simulink model "EHB_MOTOR_r2018b"  (R2018b)
settings: Solver=FixedStepDiscrete  StartTime=0.0  StopTime=0.2  FixedStep=0.0001  RelTol=1e-3  EnableMultiTasking=on
undefined symbols (not defined in the file): CAN_EHB_VCU0x125, CAN_EHB_VCU0x126, CAN_id0x120_Data, Cos_Table, Cos_Table1, EHB_DTC_status, Sin_BreakPoint, Sin_BreakPoint1, Sin_Table, Sin_Table1
libraries: simulink x30
(part 1 of 7)
settings Model: Creator=dell  LastModifiedBy=Administrator
settings SolverCC: PositivePriorityOrder=on  AutoInsertRateTranBlk=on
settings DataIOCC: LimitDataPoints=on  SaveFormat=Structure
settings OptimizationCC: DefaultParameterBehavior=Inlined  UseDivisionForNetSlopeComputation=on  InlineInvariantSignals=on  ExpressionDepthLimit=2147483647  ZeroExternalMemoryAtStartup=off  NoFixptDivByZeroProtection=on  EfficientFloat2IntCast=on  LifeSpan=1  MaxStackSize=64
settings DebuggingCC: CheckSSInitialOutputMsg=off  UnderspecifiedInitializationDetection=Classic  MergeDetectMultiDrivingBlocksExec=none  SignalResolutionControl=TryResolveAll  SolverPrmCheckMsg=warning  ParameterOverflowMsg=none  ParameterPrecisionLossMsg=none  FcnCallInpInsideContextMsg=warning  AssertControl=EnableAll  StateNameClashWarn=warning  SFUnexpectedBacktrackingDiag=warning  SFNoUnconditionalDefaultTransitionDiag=warning  SFExecutionAtInitializationDiag=none
settings HardwareCC: ProdBitPerPointer=32  ProdBitPerSizeT=32  ProdBitPerPtrDiffT=32  ProdLargestAtomicInteger=Integer  ProdLargestAtomicFloat=None  ProdIntDivRoundTo=Undefined  ProdEndianess=Unspecified  ProdWordSize=32  ProdHWDeviceType=Generic->32-bit Embedded Processor  TargetBitPerPointer=64  TargetBitPerSizeT=64  TargetBitPerPtrDiffT=64  TargetLargestAtomicInteger=Integer  TargetLongLongMode=on  TargetIntDivRoundTo=Zero  TargetEndianess=LittleEndian  TargetWordSize=64  TargetHWDeviceType=MATLAB Host  ProdEqTarget=off
settings ModelReferenceCC: UpdateModelReferenceTargets=IfOutOfDate  PropagateSignalLabelsOutOfModel=off
settings SFSimCC: SimUseLocalCustomCode=off  MATLABDynamicMemAlloc=off
settings SFSimCC: SimCustomHeaderCode=|
  | #define MCU_IDLE_ST     0
  | #define MCU_INIT_ST     1
  | #define MCU_START_ST    2
  | #define MCU_RUN_ST      3
  | #define MCU_FAULT_ST    4
  | #define MCU_WAIT_ST     5
  | 
  | // MCU_IDLE_ST = 0;
  | // MCU_INIT_ST = 1;
  | // MCU_START_ST = 2;
  | // MCU_RUN_ST = 3;
  | // MCU_FAULT_ST = 4;
  | // MCU_WAIT_ST = 5;
settings RTWCC: SystemTargetFile=ert.tlc  TemplateMakefile=ert_default_tmf  RTWUseLocalCustomCode=off  RTWUseSimCustomCode=on  IncludeHyperlinkInReport=on
settings RTWCC: CustomHeaderCode=|
  | #define MCU_IDLE_ST     0
  | #define MCU_INIT_ST     1
  | #define MCU_START_ST    2
  | #define MCU_RUN_ST      3
  | #define MCU_FAULT_ST    4
  | #define MCU_WAIT_ST     5
  | 
  | // MCU_IDLE_ST = 0;
  | // MCU_INIT_ST = 1;
  | // MCU_START_ST = 2;
  | // MCU_RUN_ST = 3;
  | // MCU_FAULT_ST = 4;
  | // MCU_WAIT_ST = 5;
settings CodeAppCC: GenerateComments=off  IgnoreCustomStorageClasses=off  CustomSymbolStrType=$N$R$M  SimulinkBlockComments=off  MATLABSourceComments=on  InternalIdentifier=Classic
settings ERTTargetCC: MultiwordLength=2048  IncludeFileDelimiter=UseQuote  InlinedParameterPlacement=NonHierarchical  ERTCustomFileTemplate=example_file_process.tlc  GlobalDataDefinition=InSeparateSourceFile  DataDefinitionFile=EHB_MOTOR_data.c  GlobalDataReference=InSeparateHeaderFile  ERTFilePackagingFormat=CompactWithDataFile  DataReferenceFile=EHB_MOTOR.h  ConvertIfToSwitch=off  SuppressUnreachableDefaultCases=off  IndentStyle=Allman  IndentSize=4  MemSecPackage=mpt
settings ConfigComp: CovMetricSettings=dw  CovSaveCumulativeToWorkspaceVar=on  CovSaveSingleToWorkspaceVar=on  CovExternalEMLEnable=off  CovSFcnEnable=off
settings SimscapeCC: SimscapeNormalizeSystem=off
settings ConfigurationSet: Description=SimMechanics 2G

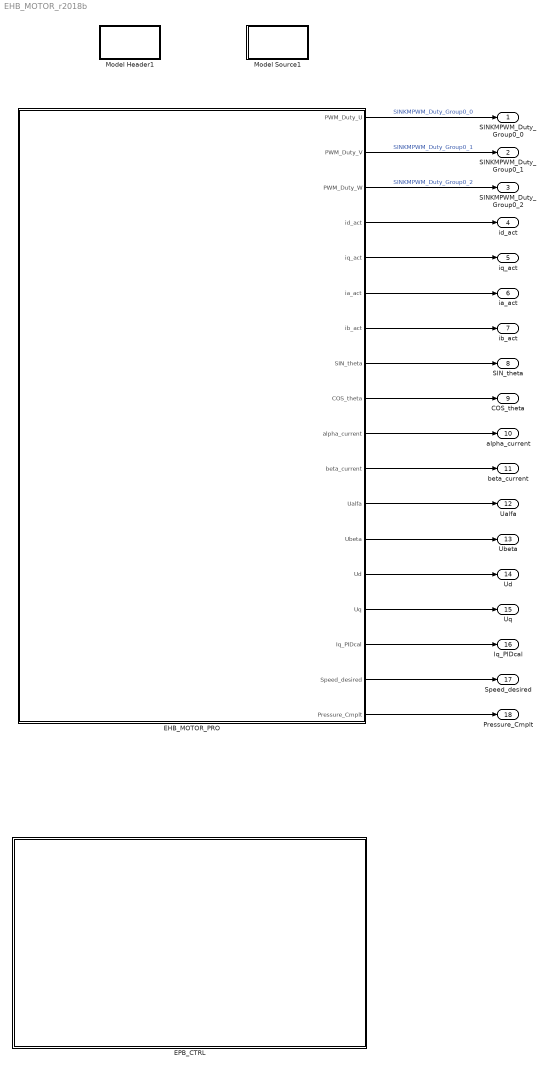
== system EHB_MOTOR_r2018b ==
  EHB_MOTOR_PRO : Subsystem  TreatAsAtomicUnit=on  RTWFcnName=isr_can_rx
      settings: MinAlgLoopOccurrences=on
  EPB_CTRL : Subsystem
  Model Header1 : Subsystem  mask(Model Header){ShowInLibBrowser=0}
      mask prompts: ShowInLibBrowser "Simulink:masks:CustCodeMaskParam1_MP"
      settings: CopyFcn=cccopyfcn(gcb)  OpenFcn=ccopenfcn('Model Header')
      mask Help: eval('feval(''rtwprivate'',''rtwhelpview'',''rtw_model_header_block'')');
      mask Display: disp('Model\nHeader');
  Model Source1 : Subsystem  mask(Model Source){ShowInLibBrowser=0}
      mask prompts: ShowInLibBrowser "Simulink:masks:CustCodeMaskParam1_MP"
      settings: CopyFcn=cccopyfcn(gcb)  OpenFcn=ccopenfcn('Model Source')
      mask Help: eval('feval(''rtwprivate'',''rtwhelpview'',''rtw_model_source_block'')');
      mask Display: disp('Model\nSource');
  SINKMPWM_Duty_Group0_0 : Outport
  SINKMPWM_Duty_Group0_1 : Outport  Port=2
  SINKMPWM_Duty_Group0_2 : Outport  Port=3
  id_act : Outport  Port=4
  iq_act : Outport  Port=5
  ia_act : Outport  Port=6
  ib_act : Outport  Port=7
  SIN_theta : Outport  Port=8
  COS_theta : Outport  Port=9
  alpha_current : Outport  Port=10  OutDataTypeStr=single
  beta_current : Outport  Port=11  OutDataTypeStr=single
  Ualfa : Outport  Port=12
  Ubeta : Outport  Port=13
  Ud : Outport  Port=14
  Uq : Outport  Port=15
  Iq_PIDcal : Outport  Port=16
  Speed_desired : Outport  Port=17
  Pressure_Cmplt : Outport  Port=18
  wires:
  EHB_MOTOR_PRO/18(Pressure_Cmplt) -> Pressure_Cmplt/1
  EHB_MOTOR_PRO/4(id_act) -> id_act/1
  EHB_MOTOR_PRO/7(ib_act) -> ib_act/1
  EHB_MOTOR_PRO/16(Iq_PIDcal) -> Iq_PIDcal/1
  EHB_MOTOR_PRO/11(beta_current) -> beta_current/1
  EHB_MOTOR_PRO/15(Uq) -> Uq/1
  EHB_MOTOR_PRO/5(iq_act) -> iq_act/1
  EHB_MOTOR_PRO/13(Ubeta) -> Ubeta/1
  EHB_MOTOR_PRO/3(PWM_Duty_W) -> SINKMPWM_Duty_Group0_2/1  "SINKMPWM_Duty_Group0_2"
  EHB_MOTOR_PRO/17(Speed_desired) -> Speed_desired/1
  EHB_MOTOR_PRO/8(SIN_theta) -> SIN_theta/1
  EHB_MOTOR_PRO/6(ia_act) -> ia_act/1
  EHB_MOTOR_PRO/9(COS_theta) -> COS_theta/1
  EHB_MOTOR_PRO/14(Ud) -> Ud/1
  EHB_MOTOR_PRO/10(alpha_current) -> alpha_current/1
  EHB_MOTOR_PRO/2(PWM_Duty_V) -> SINKMPWM_Duty_Group0_1/1  "SINKMPWM_Duty_Group0_1"
  EHB_MOTOR_PRO/12(Ualfa) -> Ualfa/1
  EHB_MOTOR_PRO/1(PWM_Duty_U) -> SINKMPWM_Duty_Group0_0/1  "SINKMPWM_Duty_Group0_0"

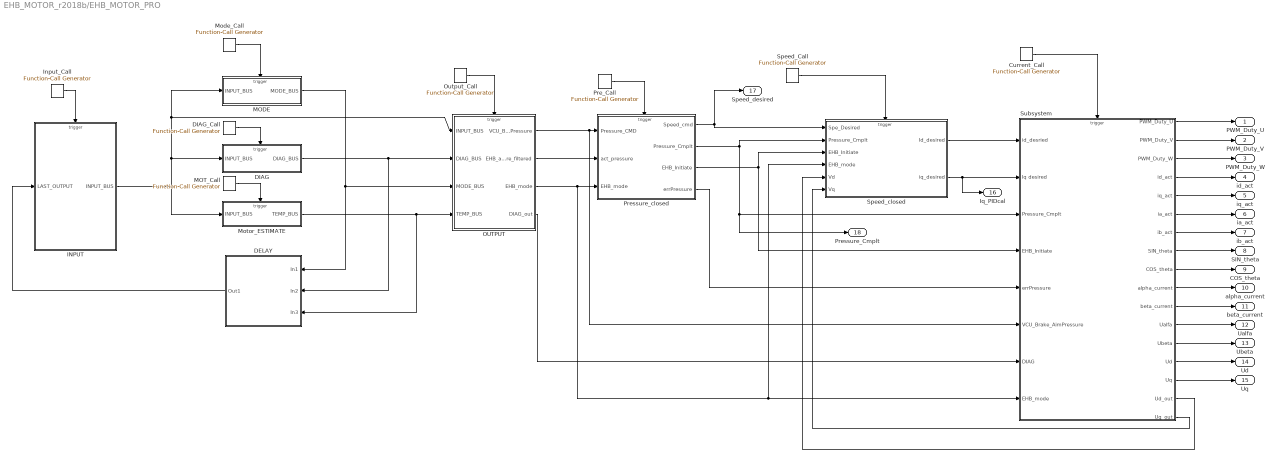
== system EHB_MOTOR_r2018b/EHB_MOTOR_PRO ==
  Current_Call : simulink/Ports & Subsystems/Function-Call Generator  sample_time=0.2  numberOfIterations=1
  DELAY : Subsystem
  DIAG : Subsystem
  DIAG_Call : simulink/Ports & Subsystems/Function-Call Generator  sample_time=0.01  numberOfIterations=1
  INPUT : Subsystem
  "Input_Call " : simulink/Ports & Subsystems/Function-Call Generator  sample_time=0.01  numberOfIterations=1
  MODE : Subsystem
  MOT_Call : simulink/Ports & Subsystems/Function-Call Generator  sample_time=0.01  numberOfIterations=1
  Mode_Call : simulink/Ports & Subsystems/Function-Call Generator  sample_time=0.01  numberOfIterations=1
  Motor_ESTIMATE : Subsystem
  OUTPUT : Subsystem
  Output_Call : simulink/Ports & Subsystems/Function-Call Generator  sample_time=0.01  numberOfIterations=1
  Pre_Call : simulink/Ports & Subsystems/Function-Call Generator  sample_time=0.05  numberOfIterations=1
  Pressure_closed : Subsystem
  "Speed_Call " : simulink/Ports & Subsystems/Function-Call Generator  sample_time=0.1  numberOfIterations=1
  Speed_closed : Subsystem
  Subsystem : Subsystem
  PWM_Duty_U : Outport
  PWM_Duty_V : Outport  Port=2
  PWM_Duty_W : Outport  Port=3
  id_act : Outport  Port=4
  iq_act : Outport  Port=5
  ia_act : Outport  Port=6  OutDataTypeStr=single
  ib_act : Outport  Port=7  OutDataTypeStr=single
  SIN_theta : Outport  Port=8
  COS_theta : Outport  Port=9
  alpha_current : Outport  Port=10  OutDataTypeStr=single
  beta_current : Outport  Port=11  OutDataTypeStr=single
  Ualfa : Outport  Port=12
  Ubeta : Outport  Port=13
  Ud : Outport  Port=14
  Uq : Outport  Port=15
  Iq_PIDcal : Outport  Port=16
  Speed_desired : Outport  Port=17
  Pressure_Cmplt : Outport  Port=18
  wires:
  "Speed_Call "/1 -> Speed_closed/Trigger
  Pressure_closed/1(Speed_cmd) -> Speed_closed/1(Spe_Desired), Speed_desired/1
  Subsystem/1(PWM_Duty_U) -> PWM_Duty_U/1
  Subsystem/2(PWM_Duty_V) -> PWM_Duty_V/1
  Subsystem/3(PWM_Duty_W) -> PWM_Duty_W/1
  Subsystem/4(id_act) -> id_act/1
  Subsystem/5(iq_act) -> iq_act/1
  Subsystem/6(ia_act) -> ia_act/1
  Subsystem/7(ib_act) -> ib_act/1
  Subsystem/8(SIN_theta) -> SIN_theta/1
  Subsystem/9(COS_theta) -> COS_theta/1
  Subsystem/10(alpha_current) -> alpha_current/1
  Subsystem/11(beta_current) -> beta_current/1
  Subsystem/12(Ualfa) -> Ualfa/1
  Subsystem/13(Ubeta) -> Ubeta/1
  Subsystem/14(Ud) -> Ud/1
  Subsystem/15(Uq) -> Uq/1
  Current_Call/1 -> Subsystem/Trigger
  Speed_closed/2(iq_desired) -> Iq_PIDcal/1, Subsystem/2(Iq desired)
  OUTPUT/1(VCU_Brake_AimPressure) -> Pressure_closed/1(Pressure_CMD), Subsystem/6(VCU_Brake_AimPressure)
  Pressure_closed/4(errPressure) -> Subsystem/5(errPressure)
  Pressure_closed/2(Pressure_Cmplt) -> Speed_closed/2(Pressure_Cmplt), Pressure_Cmplt/1, Subsystem/3(Pressure_Cmplt)
  OUTPUT/4(DIAG_out) -> Subsystem/7(DIAG)
  Pressure_closed/3(EHB_Initiate) -> Speed_closed/3(EHB_Initiate), Subsystem/4(EHB_Initiate)
  Pre_Call/1 -> Pressure_closed/Trigger
  "Input_Call "/1 -> INPUT/Trigger
  DIAG/1(DIAG_BUS) -> DELAY/2(In2), OUTPUT/2(DIAG_BUS)
  Motor_ESTIMATE/1(TEMP_BUS) -> DELAY/3(In3), OUTPUT/4(TEMP_BUS)
  MODE/1(MODE_BUS) -> DELAY/1(In1), OUTPUT/3(MODE_BUS)
  DELAY/1(Out1) -> INPUT/1(LAST_OUTPUT)
  OUTPUT/2(EHB_actPressure_filtered) -> Pressure_closed/2(act_pressure)
  INPUT/1(INPUT_BUS) -> MODE/1(INPUT_BUS), OUTPUT/1(INPUT_BUS), DIAG/1(INPUT_BUS), Motor_ESTIMATE/1(INPUT_BUS)
  Speed_closed/1(Id_desired) -> Subsystem/1(id_desried)
  Mode_Call/1 -> MODE/Trigger
  DIAG_Call/1 -> DIAG/Trigger
  Output_Call/1 -> OUTPUT/Trigger
  MOT_Call/1 -> Motor_ESTIMATE/Trigger
  OUTPUT/3(EHB_mode) -> Pressure_closed/3(EHB_mode), Speed_closed/4(EHB_mode), Subsystem/8(EHB_mode)
  Subsystem/17(Uq_out) -> Speed_closed/6(Vq)
  Subsystem/16(Ud_out) -> Speed_closed/5(Vd)

== system EHB_MOTOR_r2018b/EPB_CTRL ==
  Data Store Memory : DataStoreMemory  DataStoreName=EPB_PWMout  ReadBeforeWriteMsg=warning  WriteAfterWriteMsg=warning  WriteAfterReadMsg=warning  ShowAdditionalParam=off  OutDataTypeStr=uint16
      settings: RTWStateStorageClass=ExportedGlobal
  Data Store Memory1 : DataStoreMemory  DataStoreName=EPB_state  ReadBeforeWriteMsg=warning  WriteAfterWriteMsg=warning  WriteAfterReadMsg=warning  ShowAdditionalParam=off  OutDataTypeStr=uint8
      settings: RTWStateStorageClass=ExportedGlobal
  Data Store Memory2 : DataStoreMemory  DataStoreName=EPB_CMD  ReadBeforeWriteMsg=warning  WriteAfterWriteMsg=warning  WriteAfterReadMsg=warning  ShowAdditionalParam=off  OutDataTypeStr=uint8
      settings: RTWStateStorageClass=ExportedGlobal
  Data Store Memory3 : DataStoreMemory  DataStoreName=Clamp_ok  ReadBeforeWriteMsg=warning  WriteAfterWriteMsg=warning  WriteAfterReadMsg=warning  ShowAdditionalParam=off  OutDataTypeStr=boolean
      settings: RTWStateStorageClass=ExportedGlobal
  Data Store Memory4 : DataStoreMemory  DataStoreName=Release_ok  ReadBeforeWriteMsg=warning  WriteAfterWriteMsg=warning  WriteAfterReadMsg=warning  ShowAdditionalParam=off  OutDataTypeStr=boolean
      settings: RTWStateStorageClass=ExportedGlobal
  Data Store Read : DataStoreRead  DataStoreName=EPB_CMD  DataStoreElements=EPB_CMD
  Data Store Write : DataStoreWrite  DataStoreName=EPB_PWMout  DataStoreElements=EPB_PWMout
  Data Store Write1 : DataStoreWrite  DataStoreName=EPB_state  DataStoreElements=EPB_state
  Data Store Write2 : DataStoreWrite  DataStoreName=Clamp_ok  DataStoreElements=Clamp_ok
  Data Store Write3 : DataStoreWrite  DataStoreName=Release_ok  DataStoreElements=Release_ok
  EPBDiag_Call : simulink/Ports & Subsystems/Function-Call Generator  sample_time=0.3  numberOfIterations=1
  EPBInput_Call : simulink/Ports & Subsystems/Function-Call Generator  sample_time=0.3  numberOfIterations=1
  EPB_CTRL : Subsystem
  EPB_Diag : Subsystem
  EPBctrl_Call : simulink/Ports & Subsystems/Function-Call Generator  sample_time=0.3  numberOfIterations=1
  Subsystem1 : Subsystem
  wires:
  EPB_Diag/1(EPB_DiagBUS) -> EPB_CTRL/2(EPB_DiagBUS)
  Subsystem1/1(EPB_INPUTBUS) -> EPB_Diag/1(In1), EPB_CTRL/3(EPB_INPUTBUS)
  EPBInput_Call/1 -> Subsystem1/Trigger
  EPB_CTRL/2(EPB_state) -> Data Store Write1/1
  EPB_CTRL/4(Release_ok) -> Data Store Write3/1
  EPBctrl_Call/1 -> EPB_CTRL/Trigger
  EPB_CTRL/1(EPB_PWMout) -> Data Store Write/1
  Data Store Read/1 -> EPB_CTRL/1(EPB_CMD)
  EPB_CTRL/3(Clamp_ok) -> Data Store Write2/1
  EPBDiag_Call/1 -> EPB_Diag/Trigger

== system EHB_MOTOR_r2018b/Model Header1 ==

== system EHB_MOTOR_r2018b/Model Source1 ==

== system EHB_MOTOR_r2018b/EHB_MOTOR_PRO/DELAY ==
  In1 : Inport
  In2 : Inport  Port=2
  In3 : Inport  Port=3
  Bus Creator : BusCreator  Inputs=3
  Unit Delay : UnitDelay  SampleTime=-1
  Unit Delay1 : UnitDelay  SampleTime=-1
  Unit Delay2 : UnitDelay  SampleTime=-1
  Out1 : Outport
  wires:
  In1/1 -> Unit Delay/1
  In2/1 -> Unit Delay1/1
  Unit Delay/1 -> Bus Creator/1  "MODE_DELAY"
  Unit Delay1/1 -> Bus Creator/2  "DIAG_DELAY"
  Unit Delay2/1 -> Bus Creator/3  "TEMP_DELAY"
  Bus Creator/1 -> Out1/1
  In3/1 -> Unit Delay2/1

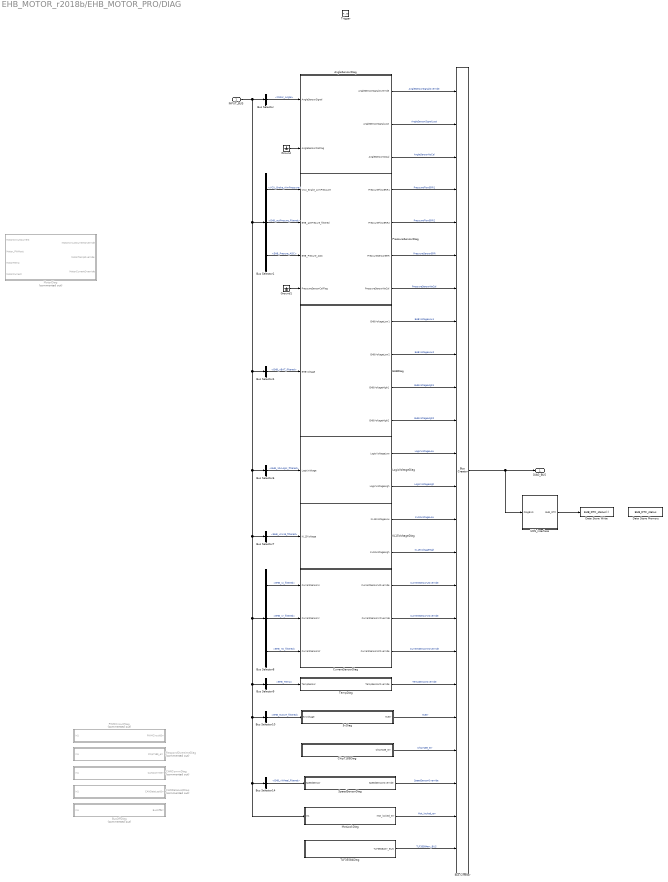
== system EHB_MOTOR_r2018b/EHB_MOTOR_PRO/DIAG ==
  INPUT_BUS : Inport
  Trigger : TriggerPort  TriggerType=function-call  VariantControl=Variant  PortDimensions=1
  5vDiag : Subsystem
  AngleSensorDiag : Subsystem
  Bus Creator : BusCreator  Inputs=24
  Bus Selector : BusSelector  OutputSignals=MOT_BUS.Motor_Angle
  Bus Selector1 : BusSelector  OutputSignals=CAN_BUS.VCU_Brake_AimPressure,AI_BUS.EHB_actPresure_filtered,AI_BUS.EHB_Presure_ADC
  Bus Selector10 : BusSelector  OutputSignals=AI_BUS.EHB_5vOUT_filtered
  Bus Selector14 : BusSelector  OutputSignals=AI_BUS.EHB_vWheel_filtered
  Bus Selector4 : BusSelector  OutputSignals=AI_BUS.EHB_vBAT_filtered
  Bus Selector6 : BusSelector  OutputSignals=AI_BUS.EHB_12vLogic_filtered
  Bus Selector7 : BusSelector  OutputSignals=AI_BUS.EHB_vKL15_filtered
  Bus Selector8 : BusSelector  OutputSignals=AI_BUS.EHB_iU_filtered,AI_BUS.EHB_iV_filtered,AI_BUS.EHB_iW_filtered
  Bus Selector9 : BusSelector  OutputSignals=AI_BUS.EHB_Temp
  BusOffDiag : Subsystem  Commented=on
  CANCommDiag : Subsystem  Commented=on
  CANDataLostDiag : Subsystem  Commented=on
  Chip7189Diag : Subsystem
  CurrentSensorDiag : Subsystem
  Data Store Memory : DataStoreMemory  DataStoreName=EHB_DTC_status  ReadBeforeWriteMsg=warning  WriteAfterWriteMsg=warning  WriteAfterReadMsg=warning  ShowAdditionalParam=off  OutDataTypeStr=uint8  Dimensions=50
      settings: RTWStateStorageClass=ExportedGlobal
  Data Store Write : DataStoreWrite  DataStoreName=EHB_DTC_status  DataStoreElements=EHB_DTC_status(:)
  EHBDiag : Subsystem
  Ground : Ground
  Ground1 : Ground
  KL15VoltageDiag : Subsystem
  LogicVoltageDiag : Subsystem
  MotLockDiag : Subsystem
  MotorDiag : Subsystem  Commented=on
  PWMCircuitDiag : Subsystem  Commented=on
  PressureSensorDiag : Subsystem
  RespondOvertimeDiag : Subsystem  Commented=on
  SpeedSensorDiag : Subsystem
  TLF35584Diag : Subsystem
  TempDiag : Subsystem
  UDS_interface : Subsystem
  DIAG_BUS : Outport
  wires:
  Bus Creator/1 -> DIAG_BUS/1, UDS_interface/1(DiagBUS)
  INPUT_BUS/1 -> Bus Selector14/1, MotLockDiag/1(In1), Bus Selector10/1, Bus Selector9/1, Bus Selector8/1, Bus Selector7/1, Bus Selector6/1, Bus Selector4/1, Bus Selector1/1, Bus Selector/1
  AngleSensorDiag/1(AngleSensorSignalOverride) -> Bus Creator/1  "AngleSensorSignalOverride"
  AngleSensorDiag/2(AngleSensorSignalLost) -> Bus Creator/2  "AngleSensorSignalLost"
  AngleSensorDiag/3(AngleSensorNoCal) -> Bus Creator/3  "AngleSensorNoCal"
  PressureSensorDiag/1(PressureFlowERR1) -> Bus Creator/4  "PressureFlowERR1"
  PressureSensorDiag/3(PressureSensorERR) -> Bus Creator/6  "PressureSensorERR"
  PressureSensorDiag/4(PressureSensorNoCal) -> Bus Creator/7  "PressureSensorNoCal"
  Bus Selector/1 -> AngleSensorDiag/1(AngleSensorSignal)  "<Motor_Angle>"
  Bus Selector1/2 -> PressureSensorDiag/2(EHB_actPresure_filtered)  "<EHB_actPresure_filtered>"
  EHBDiag/1(EHBVoltageLow1) -> Bus Creator/8  "EHBVoltageLow1"
  EHBDiag/3(EHBVoltageHigh1) -> Bus Creator/10  "EHBVoltageHigh1"
  Bus Selector4/1 -> EHBDiag/1(EHBVoltage)  "<EHB_vBAT_filtered>"
  LogicVoltageDiag/1(LogicVoltageLow) -> Bus Creator/12  "LogicVoltageLow"
  LogicVoltageDiag/2(LogicVoltageHigh) -> Bus Creator/13  "LogicVoltageHigh"
  Bus Selector6/1 -> LogicVoltageDiag/1(LogicVoltage)  "<EHB_12vLogic_filtered>"
  KL15VoltageDiag/1(KL15VoltageLow) -> Bus Creator/14  "KL15VoltageLow"
  KL15VoltageDiag/2(KL15VoltageHigh) -> Bus Creator/15  "KL15VoltageHigh"
  Bus Selector7/1 -> KL15VoltageDiag/1(KL15Voltage)  "<EHB_vKL15_filtered>"
  CurrentSensorDiag/1(CurrentSensorUOverride) -> Bus Creator/16  "CurrentSensorUOverride"
  CurrentSensorDiag/2(CurrentSensorVOverride) -> Bus Creator/17  "CurrentSensorVOverride"
  CurrentSensorDiag/3(CurrentSensorWOverride) -> Bus Creator/18  "CurrentSensorWOverride"
  Bus Selector8/1 -> CurrentSensorDiag/1(CurrentSensorU)  "<EHB_iU_filtered>"
  Bus Selector8/2 -> CurrentSensorDiag/2(CurrentSensorV)  "<EHB_iV_filtered>"
  TempDiag/1(TempSensorOverride) -> Bus Creator/19  "TempSensorOverride"
  Bus Selector9/1 -> TempDiag/1(TempSensor)  "<EHB_Temp>"
  Bus Selector10/1 -> 5vDiag/1(5vVoltage)  "<EHB_5vOUT_filtered>"
  5vDiag/1(5vErr) -> Bus Creator/20  "5vErr"
  Chip7189Diag/1(Chip7189_err) -> Bus Creator/21  "Chip7189_err"
  SpeedSensorDiag/1(SpeedSensorOverride) -> Bus Creator/22  "SpeedSensorOverride"
  Bus Selector14/1 -> SpeedSensorDiag/1(SpeedSensor)  "<EHB_vWheel_filtered>"
  Ground/1 -> AngleSensorDiag/2(AngleSensorCalFlag)
  Ground1/1 -> PressureSensorDiag/4(PressureSensorCalFlag)
  Bus Selector8/3 -> CurrentSensorDiag/3(CurrentSensorW)  "<EHB_iW_filtered>"
  Bus Selector1/1 -> PressureSensorDiag/1(VCU_Brake_AimPressure)  "<VCU_Brake_AimPressure>"
  PressureSensorDiag/2(PressureFlowERR2) -> Bus Creator/5  "PressureFlowERR2"
  EHBDiag/2(EHBVoltageLow2) -> Bus Creator/9  "EHBVoltageLow2"
  EHBDiag/4(EHBVoltageHigh2) -> Bus Creator/11  "EHBVoltageHigh2"
  MotLockDiag/1(Mot_locked_err) -> Bus Creator/23  "Mot_locked_err"
  Bus Selector1/3 -> PressureSensorDiag/3(EHB_Presure_ADC)  "<EHB_Presure_ADC>"
  UDS_interface/1(EHB_DTC) -> Data Store Write/1
  TLF35584Diag/1(TLF35584err_BUS) -> Bus Creator/24  "TLF35584err_BUS"

== system EHB_MOTOR_r2018b/EHB_MOTOR_PRO/INPUT ==
  LAST_OUTPUT : Inport
  Trigger : TriggerPort  TriggerType=function-call  VariantControl=Variant  PortDimensions=1
  AI : Subsystem
  Bus Creator : BusCreator  Inputs=5
  Bus Creator1 : BusCreator  Inputs=16
  Bus Creator2 : BusCreator  Inputs=5
  Bus Creator3 : BusCreator  Inputs=2
  Bus Creator4 : BusCreator  Inputs=10
  CAN : Subsystem
  DI : Subsystem
  MOTOR : Subsystem
  OUTPUT2INPUT : Subsystem
  INPUT_BUS : Outport
  wires:
  CAN/1(VCU_BrakingEnable) -> Bus Creator/1  "VCU_BrakingEnable"
  CAN/2(VCU_ParkingBrakeActive) -> Bus Creator/2  "VCU_ParkingBrakeActive"
  CAN/3(VCU_Brake_AimPressure) -> Bus Creator/3  "VCU_Brake_AimPressure"
  CAN/4(VCU_RollingCounter) -> Bus Creator/4  "VCU_RollingCounter"
  CAN/5(VCU_Checksum) -> Bus Creator/5  "VCU_Checksum"
  AI/1(EHB_vBAT_filtered) -> Bus Creator1/1  "EHB_vBAT_filtered"
  MOTOR/1(Motor_Angle) -> Bus Creator3/1  "Motor_Angle"
  Bus Creator/1 -> Bus Creator2/4  "CAN_BUS"
  AI/3(EHB_5vOUT_filtered) -> Bus Creator1/3  "EHB_5vOUT_filtered"
  MOTOR/2(Motor_actPWM) -> Bus Creator3/2  "Motor_actPWM"
  Bus Creator3/1 -> Bus Creator2/3  "MOT_BUS"
  LAST_OUTPUT/1 -> OUTPUT2INPUT/1(LAST_OUTPUT)
  AI/2(EHB_vKL15_filtered) -> Bus Creator1/2  "EHB_vKL15_filtered"
  AI/7(EHB_iU_filtered) -> Bus Creator1/7  "EHB_iU_filtered"
  AI/9(EHB_iV_filtered) -> Bus Creator1/9  "EHB_iV_filtered"
  AI/11(EHB_iW_filtered) -> Bus Creator1/11  "EHB_iW_filtered"
  AI/13(EHB_vWheel_filtered) -> Bus Creator1/13  "EHB_vWheel_filtered"
  DI/1(EHB_Ignion) -> Bus Creator4/1  "EHB_Ignion"
  DI/2(EHB_35584err1) -> Bus Creator4/2  "EHB_35584err1"
  DI/3(EHB_35584err2) -> Bus Creator4/3  "EHB_35584err2"
  DI/4(EHB_35584INT) -> Bus Creator4/4  "EHB_35584INT"
  DI/5(EHB_swBrkLED) -> Bus Creator4/5  "EHB_swBrkLED"
  DI/6(EHB_posLiq) -> Bus Creator4/6  "EHB_posLiq"
  DI/7(EHB_7189err1) -> Bus Creator4/7  "EHB_7189err1"
  DI/8(EHB_7189err2) -> Bus Creator4/8  "EHB_7189err2"
  DI/9(EHB_HID) -> Bus Creator4/9  "EHB_HID"
  DI/10(EHB_AVH) -> Bus Creator4/10  "EHB_AVH"
  Bus Creator4/1 -> Bus Creator2/2  "DI_BUS"
  AI/14(EHB_Reserve_filtered) -> Bus Creator1/14  "EHB_Reserve_filtered"
  AI/15(EHB_12vLogic_filtered) -> Bus Creator1/15  "EHB_12vLogic_filtered"
  AI/16(EHB_pwrPressure_filtered) -> Bus Creator1/16  "EHB_pwrPressure_filtered"
  OUTPUT2INPUT/1(Feedback) -> Bus Creator2/5  "Feedback"
  AI/8(EHB_iU_AD) -> Bus Creator1/8  "EHB_iU_AD"
  AI/10(EHB_iV_AD) -> Bus Creator1/10  "EHB_iV_AD"
  AI/12(EHB_iW_AD) -> Bus Creator1/12  "EHB_iW_AD"
  AI/5(EHB_Presure_ADC) -> Bus Creator1/5  "EHB_Presure_ADC"
  Bus Creator2/1 -> INPUT_BUS/1
  AI/4(EHB_Temp) -> Bus Creator1/4  "EHB_Temp"
  AI/6(EHB_actPresure_filtered) -> Bus Creator1/6  "EHB_actPresure_filtered"
  Bus Creator1/1 -> Bus Creator2/1  "AI_BUS"

== system EHB_MOTOR_r2018b/EHB_MOTOR_PRO/MODE ==
  note: 待增加自检类故障
  INPUT_BUS : Inport
  Trigger : TriggerPort  TriggerType=function-call  VariantControl=Variant  PortDimensions=1
  Bus Creator : BusCreator  Inputs=9
  Bus Selector : BusSelector  OutputSignals=CAN_BUS.VCU_BrakingEnable
  Bus Selector1 : BusSelector  OutputSignals=AI_BUS.EHB_iU_AD,AI_BUS.EHB_iV_AD,AI_BUS.EHB_iW_AD
  Bus Selector2 : BusSelector  OutputSignals=MOT_BUS.Motor_Angle
  Chart : Stateflow chart  TreatAsAtomicUnit=on
  Chart1 : Stateflow chart  TreatAsAtomicUnit=on
  Constant : Constant  OutDataTypeStr=uint8
  Constant1 : Constant  OutDataTypeStr=boolean
  Constant2 : Constant
  Constant3 : Constant
  Data Store Memory : DataStoreMemory  DataStoreName=ZeroCal_Flash_ok  ReadBeforeWriteMsg=warning  WriteAfterWriteMsg=warning  WriteAfterReadMsg=warning  ShowAdditionalParam=off  OutDataTypeStr=boolean
      settings: RTWStateStorageClass=ExportedGlobal
  Data Store Memory1 : DataStoreMemory  DataStoreName=Zero_Angle  ReadBeforeWriteMsg=warning  WriteAfterWriteMsg=warning  WriteAfterReadMsg=warning  ShowAdditionalParam=off  OutDataTypeStr=uint16
      settings: RTWStateStorageClass=ExportedGlobal
  Data Store Memory2 : DataStoreMemory  DataStoreName=ZeroCal_cmplt  ReadBeforeWriteMsg=warning  WriteAfterWriteMsg=warning  WriteAfterReadMsg=warning  ShowAdditionalParam=off  OutDataTypeStr=boolean
      settings: RTWStateStorageClass=ExportedGlobal
  Data Store Memory3 : DataStoreMemory  DataStoreName=ZeroCal_Req  ReadBeforeWriteMsg=warning  WriteAfterWriteMsg=warning  WriteAfterReadMsg=warning  ShowAdditionalParam=off  OutDataTypeStr=uint8
      settings: RTWStateStorageClass=ExportedGlobal
  Data Store Read : DataStoreRead  DataStoreName=ZeroCal_Flash_ok  DataStoreElements=ZeroCal_Flash_ok
  Data Store Write1 : DataStoreWrite  DataStoreName=Zero_Angle  DataStoreElements=Zero_Angle
  Data Store Write2 : DataStoreWrite  DataStoreName=ZeroCal_cmplt  DataStoreElements=ZeroCal_cmplt
  Data Store Write3 : DataStoreWrite  DataStoreName=ZeroCal_Req  DataStoreElements=ZeroCal_Req
  KL15_condition : Subsystem
  Relational Operator : RelationalOperator  Operator===  OutDataTypeStr=boolean  RndMeth=Simplest
  Relational Operator1 : RelationalOperator  Operator===  OutDataTypeStr=boolean  RndMeth=Simplest
  Subsystem : Subsystem
  Switch : Switch  Criteria=u2 ~= 0
  Unit Delay : UnitDelay  SampleTime=-1
  MODE_BUS : Outport
  wires:
  Bus Creator/1 -> MODE_BUS/1
  INPUT_BUS/1 -> Subsystem/1(INPUT_BUS), Bus Selector2/1, Bus Selector/1, Bus Selector1/1, KL15_condition/1(INPUT_BUS)
  KL15_condition/1(ignition_status) -> Chart/1(ignition)
  Bus Selector/1 -> Chart/5(EHB_mode_req)  "<VCU_BrakingEnable>"
  Chart/1(EHB_35584_en) -> Bus Creator/1  "EHB_35584_en"
  Chart/2(EHB_5vOUT_en) -> Bus Creator/2  "EHB_5vOUT_en"
  Chart/3(EHB_7189_en) -> Bus Creator/3  "EHB_7189_en"
  Chart/4(EHB_CAN_en) -> Bus Creator/4  "EHB_CAN_en"
  Chart/5(EHB_mode) -> Bus Creator/5  "EHB_mode"
  Subsystem/1(Fault_Status) -> Chart/7(Fault_Sts)
  Bus Selector1/1 -> Chart/2(Motor_iUzero_AD)  "<EHB_iU_AD>"
  Bus Selector1/2 -> Chart/3(Motor_iVzero_AD)  "<EHB_iV_AD>"
  Bus Selector1/3 -> Chart/4(Motor_iWzero_AD)  "<EHB_iW_AD>"
  Chart/6(Flash_Ucurrent) -> Bus Creator/6  "Flash_Ucurrent"
  Chart/7(Flash_Vcurrent) -> Bus Creator/7  "Flash_Vcurrent"
  Chart/8(Flash_Wcurrent) -> Bus Creator/8  "Flash_Wcurrent"
  Chart/9(EHB_AngleZeroCal_Req) -> Bus Creator/9, Relational Operator/1, Data Store Write3/1  "EHB_AngleZeroCal_Req"
  Chart1/2(ZeroCal_cmplt) -> Data Store Write2/1, Unit Delay/1
  Constant/1 -> Chart/6(Self_Check_Sts)
  Relational Operator/1 -> Chart1/2(input)
  Constant2/1 -> Relational Operator/2
  Chart1/1(Zero_Angle) -> Data Store Write1/1
  Bus Selector2/1 -> Chart1/1(MOT_Angle)  "<Motor_Angle>"
  Unit Delay/1 -> Switch/3
  Switch/1 -> Chart/8(ZeroCal_write_ok)
  Constant1/1 -> Switch/1
  Relational Operator1/1 -> Switch/2
  Data Store Read/1 -> Relational Operator1/1
  Constant3/1 -> Relational Operator1/2

== system EHB_MOTOR_r2018b/EHB_MOTOR_PRO/Motor_ESTIMATE ==
  INPUT_BUS : Inport
  Trigger : TriggerPort  TriggerType=function-call  VariantControl=Variant  PortDimensions=1
  Bus Creator : BusCreator  Inputs=2
  Bus Selector : BusSelector  OutputSignals=AI_BUS.EHB_Temp
  Bus Selector1 : BusSelector  OutputSignals=MOT_BUS.Motor_Angle
  Motor_Length : Subsystem
  Motor_Temp : Subsystem
  TEMP_BUS : Outport
  wires:
  Motor_Temp/1(EHB_Mot_temp) -> Bus Creator/1  "EHB_Mot_temp"
  Motor_Length/1(EHB_Mot_length) -> Bus Creator/2  "EHB_Mot_length"
  Bus Creator/1 -> TEMP_BUS/1
  INPUT_BUS/1 -> Bus Selector1/1, Bus Selector/1
  Bus Selector/1 -> Motor_Temp/1(In1)  "<EHB_Temp>"
  Bus Selector1/1 -> Motor_Length/1(In1)  "<Motor_Angle>"

== system EHB_MOTOR_r2018b/EHB_MOTOR_PRO/OUTPUT ==
  INPUT_BUS : Inport
  DIAG_BUS : Inport  Port=2
  MODE_BUS : Inport  Port=3
  TEMP_BUS : Inport  Port=4
  Trigger : TriggerPort  TriggerType=function-call  VariantControl=Variant  PortDimensions=1
  CAN_pack : Subsystem
  Data Store Memory3 : DataStoreMemory  DataStoreName=CAN_EHB_VCU0x125  ReadBeforeWriteMsg=warning  WriteAfterWriteMsg=warning  WriteAfterReadMsg=warning  ShowAdditionalParam=off  OutDataTypeStr=uint8  Dimensions=8
      settings: RTWStateStorageClass=ExportedGlobal
  Data Store Memory4 : DataStoreMemory  DataStoreName=CAN_EHB_VCU0x126  ReadBeforeWriteMsg=warning  WriteAfterWriteMsg=warning  WriteAfterReadMsg=warning  ShowAdditionalParam=off  OutDataTypeStr=uint8  Dimensions=8
      settings: RTWStateStorageClass=ExportedGlobal
  Data Store Write2 : DataStoreWrite  DataStoreName=CAN_EHB_VCU0x125  DataStoreElements=CAN_EHB_VCU0x125(:)
  Data Store Write3 : DataStoreWrite  DataStoreName=CAN_EHB_VCU0x126  DataStoreElements=CAN_EHB_VCU0x126(:)
  FUALT_HANDLE : Subsystem
  VCU_Brake_AimPressure : Outport
  EHB_actPressure_filtered : Outport  Port=2
  EHB_mode : Outport  Port=3
  DIAG_out : Outport  Port=4
  wires:
  INPUT_BUS/1 -> FUALT_HANDLE/1(INPUT_BUS), CAN_pack/1(INPUT_BUS)
  FUALT_HANDLE/2(EHB_actPressure_filtered) -> EHB_actPressure_filtered/1
  DIAG_BUS/1 -> FUALT_HANDLE/3(DIAG_BUS), CAN_pack/3(DIAG_BUS)
  TEMP_BUS/1 -> FUALT_HANDLE/4(TEMP_BUS)
  MODE_BUS/1 -> FUALT_HANDLE/2(MODE_BUS), CAN_pack/2(MODE_BUS)
  FUALT_HANDLE/1(VCU_Brake_AimPressure) -> VCU_Brake_AimPressure/1
  CAN_pack/1(EHB_VCU_0x125) -> Data Store Write2/1
  CAN_pack/2(EHB_VCU_0x126) -> Data Store Write3/1
  FUALT_HANDLE/4(DIAG_out) -> DIAG_out/1
  FUALT_HANDLE/3(EHB_mode) -> EHB_mode/1

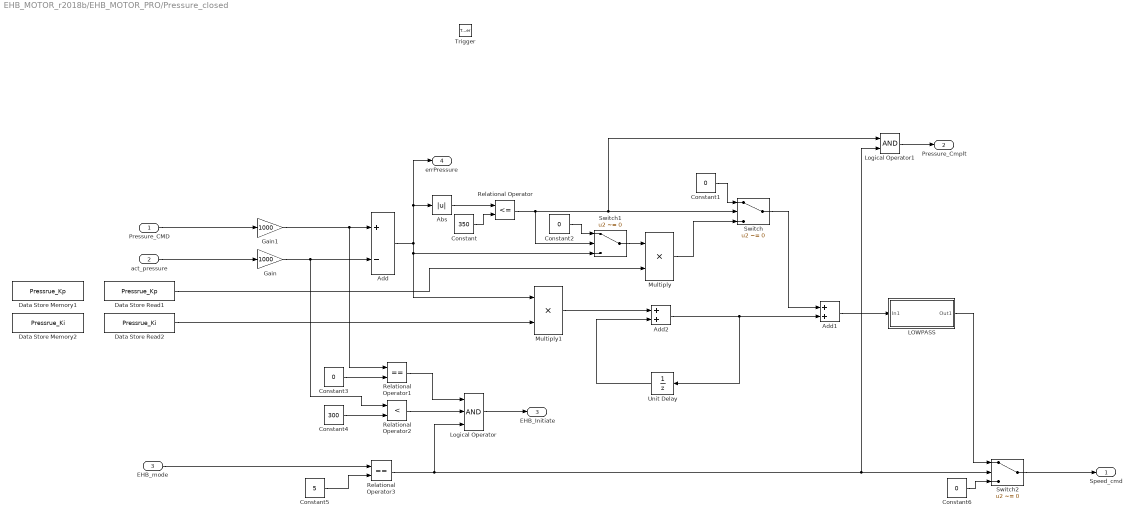
== system EHB_MOTOR_r2018b/EHB_MOTOR_PRO/Pressure_closed ==
  Pressure_CMD : Inport
  act_pressure : Inport  Port=2
  EHB_mode : Inport  Port=3
  Trigger : TriggerPort  TriggerType=function-call  VariantControl=Variant  PortDimensions=1
  Abs : Abs
  Add : Sum  Inputs=+-
  Add1 : Sum
  Add2 : Sum
  Constant : Constant  Value=350
  Constant1 : Constant  Value=0  OutDataTypeStr=single
  Constant2 : Constant  Value=0  OutDataTypeStr=single
  Constant3 : Constant  Value=0
  Constant4 : Constant  Value=300
  Constant5 : Constant  Value=5
  Constant6 : Constant  Value=0  OutDataTypeStr=single
  Data Store Memory1 : DataStoreMemory  DataStoreName=Pressrue_Kp  ReadBeforeWriteMsg=warning  WriteAfterWriteMsg=warning  WriteAfterReadMsg=warning  ShowAdditionalParam=off  OutDataTypeStr=single
      settings: RTWStateStorageClass=ExportedGlobal
  Data Store Memory2 : DataStoreMemory  DataStoreName=Pressrue_Ki  ReadBeforeWriteMsg=warning  WriteAfterWriteMsg=warning  WriteAfterReadMsg=warning  ShowAdditionalParam=off  OutDataTypeStr=single
      settings: RTWStateStorageClass=ExportedGlobal
  Data Store Read1 : DataStoreRead  DataStoreName=Pressrue_Kp  DataStoreElements=Pressrue_Kp
  Data Store Read2 : DataStoreRead  DataStoreName=Pressrue_Ki  DataStoreElements=Pressrue_Ki
  Gain : Gain  Gain=1000  OutDataTypeStr=single
  Gain1 : Gain  Gain=1000  OutDataTypeStr=single
  LOWPASS : Subsystem
  Logical Operator : Logic  Inputs=3  AllPortsSameDT=off  OutDataTypeStr=boolean
  Logical Operator1 : Logic  AllPortsSameDT=off  OutDataTypeStr=boolean
  Multiply : Product
  Multiply1 : Product
  Relational Operator : RelationalOperator  Operator=<=  OutDataTypeStr=boolean  RndMeth=Simplest
  Relational Operator1 : RelationalOperator  Operator===  OutDataTypeStr=boolean  RndMeth=Simplest
  Relational Operator2 : RelationalOperator  Operator=<  OutDataTypeStr=boolean  RndMeth=Simplest
  Relational Operator3 : RelationalOperator  Operator===  OutDataTypeStr=boolean  RndMeth=Simplest
  Switch : Switch  Criteria=u2 ~= 0
  Switch1 : Switch  Criteria=u2 ~= 0
  Switch2 : Switch  Criteria=u2 ~= 0
  Unit Delay : UnitDelay  SampleTime=-1
  Speed_cmd : Outport
  Pressure_Cmplt : Outport  Port=2
  EHB_Initiate : Outport  Port=3
  errPressure : Outport  Port=4
  wires:
  Pressure_CMD/1 -> Gain1/1
  Gain1/1 -> Add/1, Relational Operator1/1
  Gain/1 -> Add/2, Relational Operator2/1
  Data Store Read1/1 -> Multiply/2
  Add1/1 -> LOWPASS/1(In1)
  Data Store Read2/1 -> Multiply1/2
  Multiply1/1 -> Add2/1
  Add2/1 -> Unit Delay/1, Add1/2
  Unit Delay/1 -> Add2/2
  Multiply/1 -> Switch/3
  Abs/1 -> Relational Operator/1
  Constant/1 -> Relational Operator/2
  Relational Operator/1 -> Logical Operator1/1, Switch/2, Switch1/2
  Switch/1 -> Add1/1
  Constant1/1 -> Switch/1
  LOWPASS/1(Out1) -> Switch2/1
  Switch1/1 -> Multiply/1
  Constant2/1 -> Switch1/1
  Add/1 -> Switch1/3, Multiply1/1, Abs/1, errPressure/1
  Constant3/1 -> Relational Operator1/2
  Constant4/1 -> Relational Operator2/2
  Relational Operator2/1 -> Logical Operator/2
  Relational Operator1/1 -> Logical Operator/1
  Logical Operator/1 -> EHB_Initiate/1
  act_pressure/1 -> Gain/1
  EHB_mode/1 -> Relational Operator3/1
  Constant5/1 -> Relational Operator3/2
  Relational Operator3/1 -> Logical Operator/3, Switch2/2, Logical Operator1/2
  Switch2/1 -> Speed_cmd/1
  Constant6/1 -> Switch2/3
  Logical Operator1/1 -> Pressure_Cmplt/1

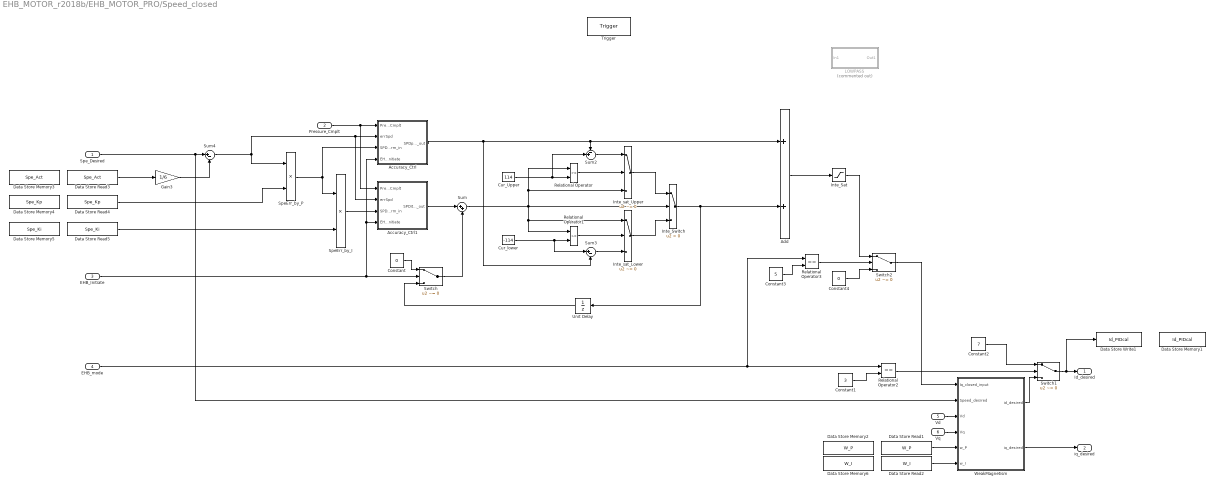
== system EHB_MOTOR_r2018b/EHB_MOTOR_PRO/Speed_closed ==
  Spe_Desired : Inport  OutDataTypeStr=single
  Pressure_Cmplt : Inport  Port=2
  EHB_Initiate : Inport  Port=3
  EHB_mode : Inport  Port=4
  Vd : Inport  Port=5
  Vq : Inport  Port=6
  Trigger : TriggerPort  TriggerType=function-call  VariantControl=(inherit)  PortDimensions=1
  Accuracy_Ctrl : Subsystem
  Accuracy_Ctrl1 : Subsystem
  Add : Sum  OutDataTypeStr=single
  Constant : Constant  Value=0
  Constant1 : Constant  Value=3
  Constant2 : Constant  Value=7  OutDataTypeStr=single
  Constant3 : Constant  Value=5
  Constant4 : Constant  Value=0  OutDataTypeStr=single
  Cur_Upper : Constant  Value=114  OutDataTypeStr=single
  Cur_lower : Constant  Value=-114  OutDataTypeStr=single
  Data Store Memory1 : DataStoreMemory  DataStoreName=Id_PIDcal  ReadBeforeWriteMsg=warning  WriteAfterWriteMsg=warning  WriteAfterReadMsg=warning  ShowAdditionalParam=off  OutDataTypeStr=single
      settings: RTWStateStorageClass=ExportedGlobal
  Data Store Memory2 : DataStoreMemory  DataStoreName=W_P  ReadBeforeWriteMsg=warning  WriteAfterWriteMsg=warning  WriteAfterReadMsg=warning  ShowAdditionalParam=off  OutDataTypeStr=single
      settings: RTWStateStorageClass=ExportedGlobal
  Data Store Memory3 : DataStoreMemory  DataStoreName=Spe_Act  ReadBeforeWriteMsg=warning  WriteAfterWriteMsg=warning  WriteAfterReadMsg=warning  ShowAdditionalParam=off  OutDataTypeStr=int16
      settings: RTWStateStorageClass=ExportedGlobal
  Data Store Memory4 : DataStoreMemory  DataStoreName=Spe_Kp  ReadBeforeWriteMsg=warning  WriteAfterWriteMsg=warning  WriteAfterReadMsg=warning  ShowAdditionalParam=off  OutDataTypeStr=single
      settings: RTWStateStorageClass=ExportedGlobal
  Data Store Memory5 : DataStoreMemory  DataStoreName=Spe_Ki  ReadBeforeWriteMsg=warning  WriteAfterWriteMsg=warning  WriteAfterReadMsg=warning  ShowAdditionalParam=off  OutDataTypeStr=single
      settings: RTWStateStorageClass=ExportedGlobal
  Data Store Memory6 : DataStoreMemory  DataStoreName=W_I  ReadBeforeWriteMsg=warning  WriteAfterWriteMsg=warning  WriteAfterReadMsg=warning  ShowAdditionalParam=off  OutDataTypeStr=single
      settings: RTWStateStorageClass=ExportedGlobal
  Data Store Read1 : DataStoreRead  DataStoreName=W_P  DataStoreElements=W_P
  Data Store Read2 : DataStoreRead  DataStoreName=W_I  DataStoreElements=W_I
  Data Store Read3 : DataStoreRead  DataStoreName=Spe_Act  DataStoreElements=Spe_Act
  Data Store Read4 : DataStoreRead  DataStoreName=Spe_Kp  DataStoreElements=Spe_Kp
  Data Store Read5 : DataStoreRead  DataStoreName=Spe_Ki  DataStoreElements=Spe_Ki
  Data Store Write1 : DataStoreWrite  DataStoreName=Id_PIDcal  DataStoreElements=Id_PIDcal
  Gain3 : Gain  Gain=1/6  OutDataTypeStr=single
  Inte_Sat : Saturate  UpperLimit=114  LowerLimit=-114
  Inte_Switch : Switch  Criteria=u2 > Threshold
  Inte_sat_Lower : Switch  Criteria=u2 ~= 0  OutDataTypeStr=single
  Inte_sat_Upper : Switch  Criteria=u2 ~= 0  OutDataTypeStr=single
  LOWPASS : Subsystem  Commented=on
  Relational Operator : RelationalOperator  OutDataTypeStr=boolean  RndMeth=Nearest
  Relational Operator1 : RelationalOperator  OutDataTypeStr=boolean  RndMeth=Nearest
  Relational Operator2 : RelationalOperator  Operator===  OutDataTypeStr=boolean  RndMeth=Simplest
  Relational Operator3 : RelationalOperator  Operator===  OutDataTypeStr=boolean  RndMeth=Simplest
  SpeErr_by_I : Product  OutDataTypeStr=single
  SpeErr_by_P : Product  OutDataTypeStr=single
  Sum : Sum  Inputs=|++
  Sum2 : Sum  Inputs=-+|  OutDataTypeStr=single
  Sum3 : Sum  Inputs=|+-  OutDataTypeStr=single
  Sum4 : Sum  Inputs=|+-
  Switch : Switch  Criteria=u2 ~= 0
  Switch1 : Switch  Criteria=u2 ~= 0
  Switch2 : Switch  Criteria=u2 ~= 0
  Unit Delay : UnitDelay  SampleTime=-1
  WeakMagnetism : Subsystem
  Id_desired : Outport
  iq_desired : Outport  Port=2
  wires:
  Sum4/1 -> SpeErr_by_P/1, Accuracy_Ctrl1/2(errSpd), Accuracy_Ctrl/2(errSpd)
  Data Store Read4/1 -> SpeErr_by_P/2
  Data Store Read5/1 -> SpeErr_by_I/2
  Inte_Sat/1 -> Switch2/1
  Gain3/1 -> Sum4/2
  Data Store Read3/1 -> Gain3/1
  Spe_Desired/1 -> Sum4/1, WeakMagnetism/2(Speed_desired)
  Add/1 -> Inte_Sat/1
  Sum3/1 -> Inte_sat_Lower/3
  Inte_sat_Upper/1 -> Inte_Switch/1
  Cur_lower/1 -> Sum3/1, Relational Operator1/2
  Cur_Upper/1 -> Sum2/2, Relational Operator/2
  Inte_sat_Lower/1 -> Inte_Switch/3
  Relational Operator1/1 -> Inte_sat_Lower/2
  Sum/1 -> Inte_sat_Lower/1, Relational Operator1/1, Inte_Switch/2, Inte_sat_Upper/3, Relational Operator/1
  Sum2/1 -> Inte_sat_Upper/1
  Relational Operator/1 -> Inte_sat_Upper/2
  SpeErr_by_P/1 -> Accuracy_Ctrl/3(SPDpterm_in), SpeErr_by_I/1
  SpeErr_by_I/1 -> Accuracy_Ctrl1/3(SPDiterm_in)
  Accuracy_Ctrl/1(SPDpterm_out) -> Sum3/2, Sum2/1, Add/1
  Accuracy_Ctrl1/1(SPDiterm_out) -> Sum/1
  Inte_Switch/1 -> Unit Delay/1, Add/2
  Unit Delay/1 -> Switch/3
  Pressure_Cmplt/1 -> Accuracy_Ctrl1/1(Pressure_Cmplt), Accuracy_Ctrl/1(Pressure_Cmplt)
  EHB_Initiate/1 -> Switch/2, Accuracy_Ctrl1/4(EHB_Initiate), Accuracy_Ctrl/4(EHB_Initiate)
  Constant/1 -> Switch/1
  Switch/1 -> Sum/2
  EHB_mode/1 -> Relational Operator2/1, Relational Operator3/1
  Constant1/1 -> Relational Operator2/2
  Relational Operator2/1 -> Switch1/2
  Constant2/1 -> Switch1/1
  Switch1/1 -> Id_desired/1, Data Store Write1/1
  WeakMagnetism/1(id_desired) -> Switch1/3
  Relational Operator3/1 -> Switch2/2
  Constant3/1 -> Relational Operator3/2
  Switch2/1 -> WeakMagnetism/1(Iq_closed_input)
  Constant4/1 -> Switch2/3
  WeakMagnetism/2(iq_desired) -> iq_desired/1
  Data Store Read1/1 -> WeakMagnetism/5(w_P)
  Data Store Read2/1 -> WeakMagnetism/6(w_I)
  Vd/1 -> WeakMagnetism/3(Vd)
  Vq/1 -> WeakMagnetism/4(Vq)

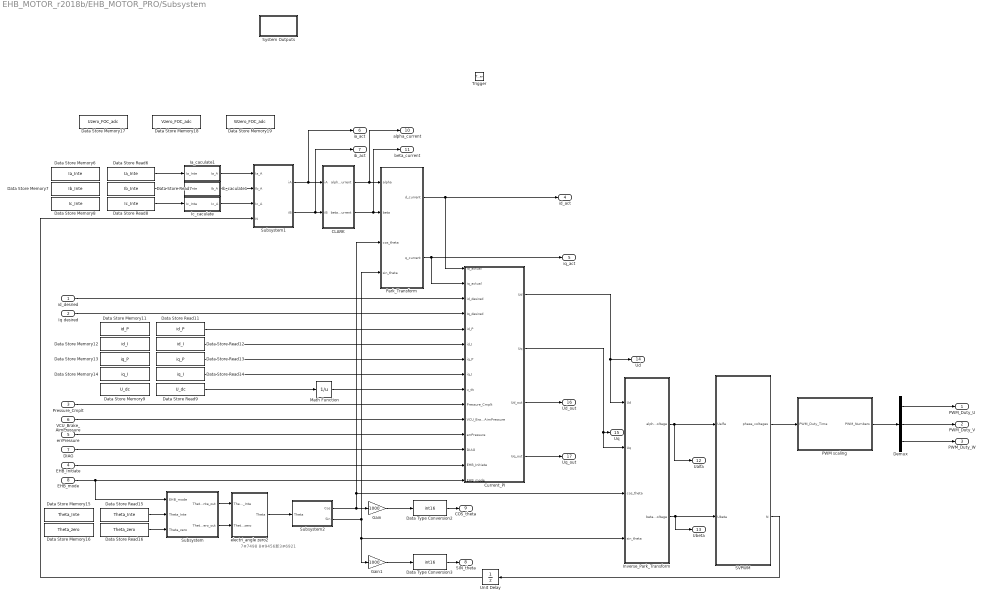
== system EHB_MOTOR_r2018b/EHB_MOTOR_PRO/Subsystem ==
  note: 7#7498
      | 8#9456
      | 新3#6921
  id_desried : Inport
  Iq desired : Inport  Port=2  OutDataTypeStr=single
  Pressure_Cmplt : Inport  Port=3
  EHB_Initiate : Inport  Port=4
  errPressure : Inport  Port=5
  VCU_Brake_AimPressure : Inport  Port=6
  DIAG : Inport  Port=7
  EHB_mode : Inport  Port=8
  Trigger : TriggerPort  TriggerType=function-call  VariantControl=Variant  PortDimensions=1
  CLARK : Subsystem
  Current_PI : Subsystem
  Data Store Memory11 : DataStoreMemory  DataStoreName=id_P  ReadBeforeWriteMsg=warning  WriteAfterWriteMsg=warning  WriteAfterReadMsg=warning  ShowAdditionalParam=off  OutDataTypeStr=single
      settings: RTWStateStorageClass=ExportedGlobal
  Data Store Memory12 : DataStoreMemory  DataStoreName=id_I  ReadBeforeWriteMsg=warning  WriteAfterWriteMsg=warning  WriteAfterReadMsg=warning  ShowAdditionalParam=off  OutDataTypeStr=single
      settings: RTWStateStorageClass=ExportedGlobal
  Data Store Memory13 : DataStoreMemory  DataStoreName=iq_P  ReadBeforeWriteMsg=warning  WriteAfterWriteMsg=warning  WriteAfterReadMsg=warning  ShowAdditionalParam=off  OutDataTypeStr=single
      settings: RTWStateStorageClass=ExportedGlobal
  Data Store Memory14 : DataStoreMemory  DataStoreName=iq_I  ReadBeforeWriteMsg=warning  WriteAfterWriteMsg=warning  WriteAfterReadMsg=warning  ShowAdditionalParam=off  OutDataTypeStr=single
      settings: RTWStateStorageClass=ExportedGlobal
  Data Store Memory15 : DataStoreMemory  DataStoreName=Theta_Inte  ReadBeforeWriteMsg=warning  WriteAfterWriteMsg=warning  WriteAfterReadMsg=warning  ShowAdditionalParam=off  OutDataTypeStr=uint16
      settings: RTWStateStorageClass=ExportedGlobal
  Data Store Memory16 : DataStoreMemory  DataStoreName=Theta_zero  ReadBeforeWriteMsg=warning  WriteAfterWriteMsg=warning  WriteAfterReadMsg=warning  ShowAdditionalParam=off  OutDataTypeStr=uint16
      settings: RTWStateStorageClass=ExportedGlobal
  Data Store Memory17 : DataStoreMemory  DataStoreName=Uzero_FOC_adc  ReadBeforeWriteMsg=warning  WriteAfterWriteMsg=warning  WriteAfterReadMsg=warning  ShowAdditionalParam=off  OutDataTypeStr=uint16
      settings: RTWStateStorageClass=ExportedGlobal
  Data Store Memory18 : DataStoreMemory  DataStoreName=Vzero_FOC_adc  ReadBeforeWriteMsg=warning  WriteAfterWriteMsg=warning  WriteAfterReadMsg=warning  ShowAdditionalParam=off  OutDataTypeStr=uint16
      settings: RTWStateStorageClass=ExportedGlobal
  Data Store Memory19 : DataStoreMemory  DataStoreName=Wzero_FOC_adc  ReadBeforeWriteMsg=warning  WriteAfterWriteMsg=warning  WriteAfterReadMsg=warning  ShowAdditionalParam=off  OutDataTypeStr=uint16
      settings: RTWStateStorageClass=ExportedGlobal
  Data Store Memory6 : DataStoreMemory  DataStoreName=Ia_Inte  ReadBeforeWriteMsg=warning  WriteAfterWriteMsg=warning  WriteAfterReadMsg=warning  ShowAdditionalParam=off  OutDataTypeStr=uint16
      settings: RTWStateStorageClass=ExportedGlobal
  Data Store Memory7 : DataStoreMemory  DataStoreName=Ib_Inte  ReadBeforeWriteMsg=warning  WriteAfterWriteMsg=warning  WriteAfterReadMsg=warning  ShowAdditionalParam=off  OutDataTypeStr=uint16
      settings: RTWStateStorageClass=ExportedGlobal
  Data Store Memory8 : DataStoreMemory  DataStoreName=Ic_Inte  ReadBeforeWriteMsg=warning  WriteAfterWriteMsg=warning  WriteAfterReadMsg=warning  ShowAdditionalParam=off  OutDataTypeStr=uint16
      settings: RTWStateStorageClass=ExportedGlobal
  Data Store Memory9 : DataStoreMemory  DataStoreName=U_dc  ReadBeforeWriteMsg=warning  WriteAfterWriteMsg=warning  WriteAfterReadMsg=warning  ShowAdditionalParam=off  OutDataTypeStr=single
      settings: RTWStateStorageClass=ExportedGlobal
  Data Store Read11 : DataStoreRead  DataStoreName=id_P  DataStoreElements=id_P
  Data Store Read12 : DataStoreRead  DataStoreName=id_I  DataStoreElements=id_I
  Data Store Read13 : DataStoreRead  DataStoreName=iq_P  DataStoreElements=iq_P
  Data Store Read14 : DataStoreRead  DataStoreName=iq_I  DataStoreElements=iq_I
  Data Store Read15 : DataStoreRead  DataStoreName=Theta_Inte  DataStoreElements=Theta_Inte
  Data Store Read16 : DataStoreRead  DataStoreName=Theta_zero  DataStoreElements=Theta_zero
  Data Store Read6 : DataStoreRead  DataStoreName=Ia_Inte  DataStoreElements=Ia_Inte
  Data Store Read7 : DataStoreRead  DataStoreName=Ib_Inte  DataStoreElements=Ib_Inte
  Data Store Read8 : DataStoreRead  DataStoreName=Ic_Inte  DataStoreElements=Ic_Inte
  Data Store Read9 : DataStoreRead  DataStoreName=U_dc  DataStoreElements=U_dc
  Data Type Conversion2 : DataTypeConversion  OutDataTypeStr=int16
  Data Type Conversion3 : DataTypeConversion  OutDataTypeStr=int16
  Demux : Demux  Outputs=3
  Gain : Gain  Gain=1000
  Gain1 : Gain  Gain=1000
  Ia_caculate1 : Subsystem
  Ib_caculate1 : Subsystem
  Ic_caculate : Subsystem
  Inverse_Park_Transform : Subsystem
  Math Function : Math  Operator=reciprocal  OutDataTypeStr=single  SaturateOnIntegerOverflow=on
  PWM scaling : Subsystem
  Park_Transform : Subsystem
  SVPWM : Subsystem
  Subsystem : Subsystem
  Subsystem1 : Subsystem
  Subsystem2 : Subsystem
  System Outputs : Subsystem  mask(System Outputs){ShowInLibBrowser=0}
      mask prompts: ShowInLibBrowser "Simulink:masks:CustCodeMaskParam1_MP"
      settings: CopyFcn=cccopyfcn(gcb)  OpenFcn=ccopenfcn('System Outputs Function')
      mask Help: eval('feval(''rtwprivate'',''rtwhelpview'',''rtw_sys_outputs_block'')');
      mask Display: disp('System\nOutputs');
  Unit Delay : UnitDelay  SampleTime=-1
  electri_angle zero2 : Subsystem
  PWM_Duty_U : Outport
  PWM_Duty_V : Outport  Port=2
  PWM_Duty_W : Outport  Port=3
  id_act : Outport  Port=4
  iq_act : Outport  Port=5
  ia_act : Outport  Port=6  OutDataTypeStr=single
  ib_act : Outport  Port=7  OutDataTypeStr=single
  SIN_theta : Outport  Port=8
  COS_theta : Outport  Port=9
  alpha_current : Outport  Port=10  OutDataTypeStr=single
  beta_current : Outport  Port=11  OutDataTypeStr=single
  Ualfa : Outport  Port=12
  Ubeta : Outport  Port=13
  Ud : Outport  Port=14
  Uq : Outport  Port=15
  Ud_out : Outport  Port=16  OutDataTypeStr=single
  Uq_out : Outport  Port=17  OutDataTypeStr=single
  wires:
  Inverse_Park_Transform/2(beta_voltage) -> Ubeta/1, SVPWM/2(Ubeta)
  Iq desired/1 -> Current_PI/4(Iq_desired)
  Data Store Read13/1 -> Current_PI/7(iq_P)
  CLARK/1(alpha_current) -> alpha_current/1, Park_Transform/1(alpha)
  Demux/1 -> PWM_Duty_U/1
  CLARK/2(beta_current) -> beta_current/1, Park_Transform/2(beta)
  Data Store Read12/1 -> Current_PI/6(id_I)
  Data Store Read14/1 -> Current_PI/8(iq_I)
  Park_Transform/2(q_current) -> Current_PI/2(iq_actual), iq_act/1
  Current_PI/2(Uq) -> Inverse_Park_Transform/2(Uq), Uq/1
  Data Store Read11/1 -> Current_PI/5(id_P)
  Math Function/1 -> Current_PI/9(u_dc)
  Gain1/1 -> Data Type Conversion3/1
  Gain/1 -> Data Type Conversion2/1
  Inverse_Park_Transform/1(alpha_voltage) -> Ualfa/1, SVPWM/1(Ualfa)
  Current_PI/1(Ud) -> Inverse_Park_Transform/1(Ud), Ud/1
  Data Type Conversion3/1 -> SIN_theta/1
  Subsystem1/1(iA) -> ia_act/1, CLARK/1(iA)
  PWM scaling/1(PWM_Numbers) -> Demux/1
  Park_Transform/1(d_current) -> Current_PI/1(id_actual), id_act/1
  Subsystem1/2(iB) -> ib_act/1, CLARK/2(iB)
  Demux/3 -> PWM_Duty_W/1
  Data Store Read7/1 -> Ib_caculate1/1(Ib_Inte)
  Data Store Read6/1 -> Ia_caculate1/1(Ia_Inte)
  Data Store Read9/1 -> Math Function/1
  Demux/2 -> PWM_Duty_V/1
  Data Type Conversion2/1 -> COS_theta/1
  id_desried/1 -> Current_PI/3(id_desired)
  SVPWM/1(phase_voltages) -> PWM scaling/1(PWM_Duty_Time)
  Pressure_Cmplt/1 -> Current_PI/10(Pressure_Cmplt)
  VCU_Brake_AimPressure/1 -> Current_PI/11(VCU_Brake_AimPressure)
  Ib_caculate1/1(Ib_A) -> Subsystem1/2(Ib_A)
  Ia_caculate1/1(Ia_A) -> Subsystem1/1(Ia_A)
  Ic_caculate/1(Ic_A) -> Subsystem1/3(Ic_A)
  Data Store Read8/1 -> Ic_caculate/1(Ic_Inte)
  SVPWM/2(N) -> Unit Delay/1
  Unit Delay/1 -> Subsystem1/4(N)
  Subsystem2/1(Cos) -> Park_Transform/3(cos_theta), Inverse_Park_Transform/3(cos_theta), Gain/1
  Subsystem2/2(Sin) -> Gain1/1, Inverse_Park_Transform/4(sin_theta), Park_Transform/4(sin_theta)
  electri_angle zero2/1(Theta) -> Subsystem2/1(Theta)
  errPressure/1 -> Current_PI/12(errPressure)
  DIAG/1 -> Current_PI/13(DIAG)
  EHB_Initiate/1 -> Current_PI/14(EHB_Initiate)
  EHB_mode/1 -> Subsystem/1(EHB_mode), Current_PI/15(EHB_mode)
  Data Store Read15/1 -> Subsystem/2(Theta_Inte)
  Data Store Read16/1 -> Subsystem/3(Theta_zero)
  Subsystem/1(Theta_Inte_out) -> electri_angle zero2/1(Theta_Inte)
  Subsystem/2(Theta_zero_out) -> electri_angle zero2/2(Theta_zero)
  Current_PI/4(Uq_out) -> Uq_out/1
  Current_PI/3(Ud_out) -> Ud_out/1

== system EHB_MOTOR_r2018b/EPB_CTRL/EPB_CTRL ==
  EPB_CMD : Inport
  EPB_DiagBUS : Inport  Port=2
  EPB_INPUTBUS : Inport  Port=3
  Trigger : TriggerPort  TriggerType=function-call  VariantControl=Variant  PortDimensions=1
  Bus Selector : BusSelector  OutputSignals=EPB1_Current_filtered,EPB2_Current_filtered
  Chart : Stateflow chart  TreatAsAtomicUnit=on
  Constant : Constant  Value=0  OutDataTypeStr=uint8
  Data Store Memory1 : DataStoreMemory  DataStoreName=EPB_tiRelease_C  ReadBeforeWriteMsg=warning  WriteAfterWriteMsg=warning  WriteAfterReadMsg=warning  ShowAdditionalParam=off  OutDataTypeStr=uint16
      settings: RTWStateStorageClass=ExportedGlobal
  Data Store Memory2 : DataStoreMemory  DataStoreName=EPB_tiClamp_C  ReadBeforeWriteMsg=warning  WriteAfterWriteMsg=warning  WriteAfterReadMsg=warning  ShowAdditionalParam=off  OutDataTypeStr=uint16
      settings: RTWStateStorageClass=ExportedGlobal
  Data Store Memory3 : DataStoreMemory  DataStoreName=EPB1_iAct_C  ReadBeforeWriteMsg=warning  WriteAfterWriteMsg=warning  WriteAfterReadMsg=warning  ShowAdditionalParam=off  OutDataTypeStr=single
      settings: RTWStateStorageClass=ExportedGlobal
  Data Store Memory4 : DataStoreMemory  DataStoreName=EPB2_iAct_C  ReadBeforeWriteMsg=warning  WriteAfterWriteMsg=warning  WriteAfterReadMsg=warning  ShowAdditionalParam=off  OutDataTypeStr=single
      settings: RTWStateStorageClass=ExportedGlobal
  Data Store Read : DataStoreRead  DataStoreName=EPB_tiClamp_C  DataStoreElements=EPB_tiClamp_C
  Data Store Read1 : DataStoreRead  DataStoreName=EPB_tiRelease_C  DataStoreElements=EPB_tiRelease_C
  Data Store Read2 : DataStoreRead  DataStoreName=EPB1_iAct_C  DataStoreElements=EPB1_iAct_C
  Data Store Read3 : DataStoreRead  DataStoreName=EPB2_iAct_C  DataStoreElements=EPB2_iAct_C
  Fault_Handle : Subsystem
  Switch : Switch  Criteria=u2 ~= 0
  EPB_PWMout : Outport
  EPB_state : Outport  Port=2
  Clamp_ok : Outport  Port=3
  Release_ok : Outport  Port=4
  wires:
  EPB_INPUTBUS/1 -> Bus Selector/1
  EPB_CMD/1 -> Chart/1(EPB_Ctrl_Req)
  Bus Selector/1 -> Chart/2(EPB1_iAct)  "<EPB1_Current_filtered>"
  Bus Selector/2 -> Chart/3(EPB2_iAct)  "<EPB2_Current_filtered>"
  Data Store Read/1 -> Chart/4(EPB_tiClamp_C)
  Data Store Read1/1 -> Chart/5(EPB_tiRelease_C)
  Data Store Read2/1 -> Chart/6(EPB1_iAct_C)
  Data Store Read3/1 -> Chart/7(EPB2_iAct_C)
  Chart/1(EPB_PWMout) -> Switch/3
  Chart/2(EPB_dir_state) -> EPB_state/1
  Chart/3(Clamp_ok) -> Clamp_ok/1
  Chart/4(Release_ok) -> Release_ok/1
  EPB_DiagBUS/1 -> Fault_Handle/1(In1)
  Fault_Handle/1(Out1) -> Switch/2
  Constant/1 -> Switch/1
  Switch/1 -> EPB_PWMout/1

== system EHB_MOTOR_r2018b/EPB_CTRL/EPB_Diag ==
  In1 : Inport
  Trigger : TriggerPort  TriggerType=function-call  VariantControl=Variant  PortDimensions=1
  Bus Creator : BusCreator  Inputs=4
  Bus Selector13 : BusSelector  OutputSignals=EPB1_Current_filtered,EPB2_Current_filtered
  Bus Selector15 : BusSelector  OutputSignals=EPB1_Temp
  Bus Selector5 : BusSelector  OutputSignals=EPB_vBAT_filtered
  EPBCurrentDiag : Subsystem
  EPBOverheatDiag : Subsystem
  EPB_vBATDiag : Subsystem
  EPB_DiagBUS : Outport
  wires:
  Bus Selector5/1 -> EPB_vBATDiag/1(EPBVoltage)  "<EPB_vBAT_filtered>"
  Bus Selector15/1 -> EPBOverheatDiag/1(EPBTemp)  "<EPB1_Temp>"
  Bus Selector13/2 -> EPBCurrentDiag/2(EPB2Current)  "<EPB2_Current_filtered>"
  Bus Selector13/1 -> EPBCurrentDiag/1(EPB1Current)  "<EPB1_Current_filtered>"
  In1/1 -> Bus Selector13/1, Bus Selector15/1, Bus Selector5/1
  EPB_vBATDiag/1(EPBVoltageLow) -> Bus Creator/1  "EPBVoltageLow"
  EPB_vBATDiag/2(EPBVoltageHigh) -> Bus Creator/2  "EPBVoltageHigh"
  EPBOverheatDiag/1(EPBOverheat) -> Bus Creator/3  "EPBOverheat"
  EPBCurrentDiag/1(EPBCurrentOverride) -> Bus Creator/4  "EPBCurrentOverride"
  Bus Creator/1 -> EPB_DiagBUS/1
